simulink model "stabilization_model"  (R2024b)
settings: Solver=ode4  StartTime=0.0  StopTime=30  FixedStep=0.0001  MaxStep=0.0005  RelTol=1e-5
values from neighbouring files (symbols this model uses):
  B_m = 0.0015    [model_consts.m]
  Bmh = 0.0015    [model_consts.m]
  C1 = 10e4    (= 100000)    [model_consts.m]
  C2 = 3    [model_consts.m]
  f_const = (4*pi^2*ni*N^2*l_1*l_2)/(p_h^2)    (= 461404.005751)    [model_consts.m]
  g1_const = (2*k_t*pi*ni*N)/(p_h*R)    (= 6268.81826761)    [model_consts.m]
  g3_const = f_const*(k_t*k_e)/(R+B_m)    (= 1536817.32754)    [model_consts.m]
  g4_const = f_const*J_m    (= 922.808011502)    [model_consts.m]
  J = 3400    [model_consts.m]
  J_m = 0.002    [model_consts.m]
  Jh = J_w + J_a + J_mw*nih*R_z*(1/R_w)    (= 26100.0000385)    [model_consts.m]
  kh_e = 0.401    [model_consts.m]
  kh_t = 0.54    [model_consts.m]
  l_1 = 0.32    [model_consts.m]
  l_2 = 0.44    [model_consts.m]
  mg = m*g    (= 19620)    [model_consts.m]
  mgl = m*g*l    (= 2354.4)    [model_consts.m]
  mwag = g*(mw+ma)    (= 186390)    [model_consts.m]
  nih = 0.97    [model_consts.m]
  q_0 = acos((l_1^2+l_2^2-l_0^2)/(2*l_1*l_2))    [model_consts.m]
  R_h = 0.01437    [model_consts.m]
  r_t = 0.05    [model_consts.m]
  R_w = 1.2    [model_consts.m]
  R_z = 0.08    [model_consts.m]
  u_k = 0.04    [model_consts.m]
  u_s = 0.12    [model_consts.m]
  uw_k = 0.0015    [model_consts.m]
  uw_s = 0.0025    [model_consts.m]
libraries: slpidlib x6, SignalEditorBlockLib x1
settings Model: Creator=ksapi  LastModifiedBy=ksapi

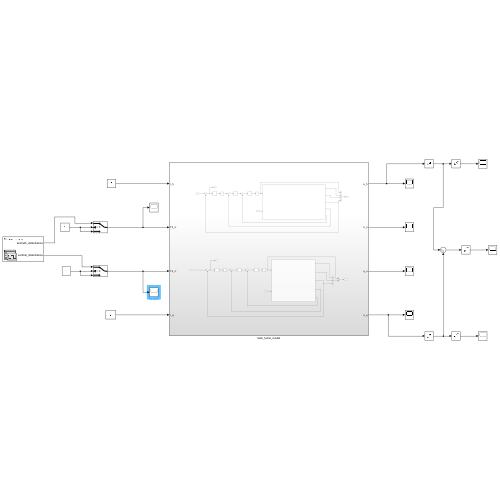
[thumbnail: Simulink's stored preview of the top-level diagram]
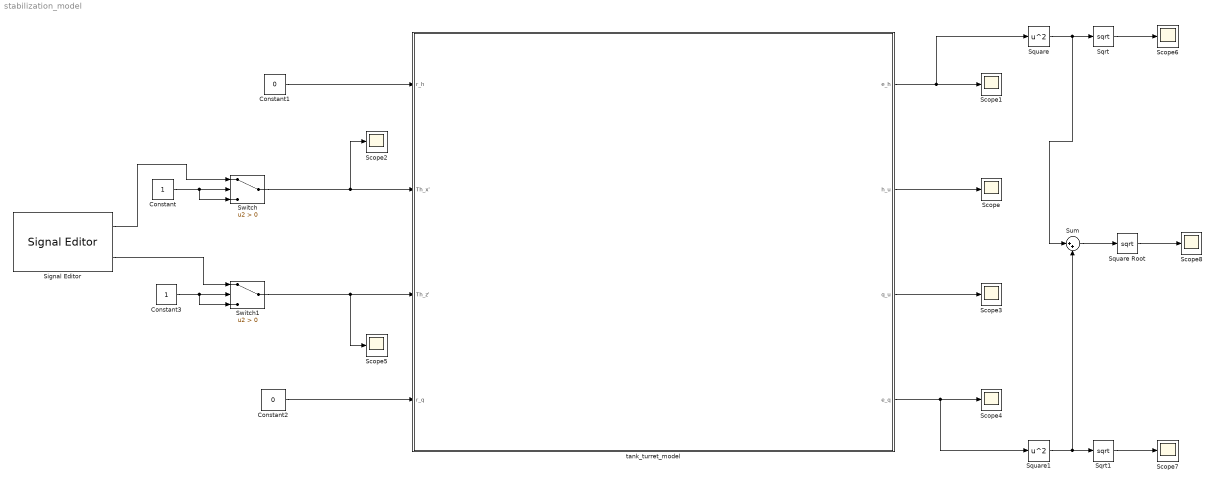
== system stabilization_model ==
  Constant : Constant
  Constant1 : Constant  Value=0
  Constant2 : Constant  Value=0
  Constant3 : Constant
  Scope{,1..8} (9 alike) : Scope
  Signal Editor : SignalEditorBlockLib/Signal Editor  FileName=disturbance_scenarios.mat  ActiveScenario=Sinous_course  ActiveSignal=azimuth_disturbance  IsBus=off  OutputBusObjectStr=Bus: BusObject  SampleTime=0  Interpolate=off  ZeroCross=off  OutputAfterFinalValue=Setting to zero  Unit=inherit  PreserveSignalName=on  ApplySigPropsToAllScenarios=on  ApplySigPropsToAllSignals=off
  Sqrt : Sqrt
  Sqrt1 : Sqrt
  Square : Math  Operator=square
  Square Root : Sqrt
  Square1 : Math  Operator=square
  Sum : Sum  Inputs=|++
  Switch : Switch  Criteria=u2 > Threshold  SaturateOnIntegerOverflow=off  InputSameDT=off
  Switch1 : Switch  Criteria=u2 > Threshold  SaturateOnIntegerOverflow=off  InputSameDT=off
  tank_turret_model : Subsystem
  wires:
  Constant1/1 -> tank_turret_model/1(r_h)
  Signal Editor/2 -> Switch1/1
  Constant2/1 -> tank_turret_model/4(r_q)
  tank_turret_model/1(e_h) -> Square/1, Scope1/1
  tank_turret_model/2(h_u) -> Scope/1
  tank_turret_model/3(q_u) -> Scope3/1
  Square/1 -> Sum/1, Sqrt/1
  Sqrt/1 -> Scope6/1
  Constant/1 -> Switch/3, Switch/2
  Constant3/1 -> Switch1/3, Switch1/2
  Signal Editor/1 -> Switch/1
  Square1/1 -> Sqrt1/1, Sum/2
  Sqrt1/1 -> Scope7/1
  tank_turret_model/4(e_q) -> Square1/1, Scope4/1
  Sum/1 -> Square Root/1
  Square Root/1 -> Scope8/1
  Switch/1 -> tank_turret_model/2(Th_x'), Scope2/1
  Switch1/1 -> tank_turret_model/3(Th_z'), Scope5/1

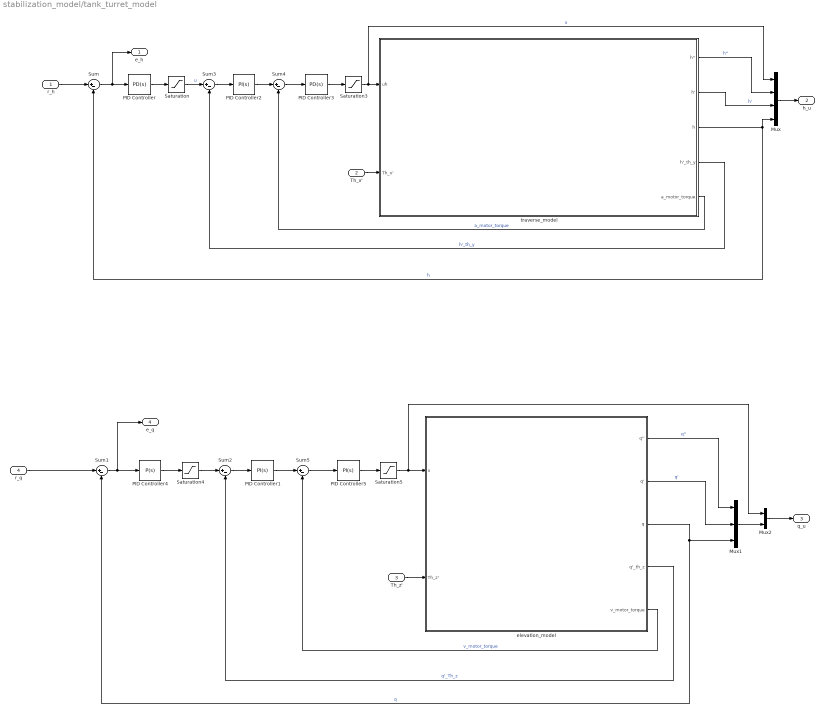
== system stabilization_model/tank_turret_model ==
  r_h : Inport
  Th_x' : Inport  Port=2
  Th_z' : Inport  Port=3
  r_q : Inport  Port=4
  Mux : Mux
  Mux1 : Mux  Inputs=3
  Mux2 : Mux  Inputs=2
  PID Controller : slpidlib/PID Controller  Controller=PD  Form=Parallel  TimeDomain=Continuous-time  UseExternalTs=off  SampleTime=-1  IntegratorMethod=Forward Euler  FilterMethod=Forward Euler  ControllerParametersSource=internal  P=140  I=0  UseKiTs=off  D=90  UseExternalDerivativeSource=off  N=100  UseFilter=on  TunerSelectOption=Transfer Function Based (PID Tuner App)  InitialConditionSource=internal  InitialConditionForIntegrator=0  InitialConditionForFilter=0  DifferentiatorICPrevScaledInput=0  ExternalReset=none  TrackingMode=off  Kt=1  LimitOutput=off  SatLimitsSource=internal  UpperSaturationLimit=inf  LowerSaturationLimit=-inf  LinearizeAsGain=on  AntiWindupMode=none  Kb=1  LimitIntegrator=off  UpperIntegratorSaturationLimit=inf  LowerIntegratorSaturationLimit=-inf  POutMin=[]  POutMax=[]  IOutMin=[]  IOutMax=[]  DOutMin=[]  DOutMax=[]  NOutMin=[]  NOutMax=[]  SumOutMin=[]  SumOutMax=[]  SaturationOutMin=[]  SaturationOutMax=[]  PParamMin=[]  PParamMax=[]  IParamMin=[]  IParamMax=[]  DParamMin=[]  DParamMax=[]  NParamMin=[]  NParamMax=[]  KbParamMin=[]  KbParamMax=[]  KtParamMin=[]  KtParamMax=[]  KbOutMin=[]  KbOutMax=[]  KtOutMin=[]  KtOutMax=[]  IntegratorOutMin=[]  IntegratorOutMax=[]  FilterOutMin=[]  FilterOutMax=[]  SumI1OutMin=[]  SumI1OutMax=[]  SumI2OutMin=[]  SumI2OutMax=[]  SumI3OutMin=[]  SumI3OutMax=[]  SumI4OutMin=[]  SumI4OutMax=[]  SumDOutMin=[]  SumDOutMax=[]  DifferentiatorOutMin=[]  DifferentiatorOutMax=[]  FilterDiffOutCoefMin=[]  FilterDiffOutCoefMax=[]  ReciprocalOutMin=[]  ReciprocalOutMax=[]  SumDenOutMin=[]  SumDenOutMax=[]  SumNumOutMin=[]  SumNumOutMax=[]  DivideOutMin=[]  DivideOutMax=[]  UdiffTsProdOutMin=[]  UdiffTsProdOutMax=[]  NTsProdOutMin=[]  NTsProdOutMax=[]  UintegralTsProdOutMin=[]  UintegralTsProdOutMax=[]  UngainTsProdOutMin=[]  UngainTsProdOutMax=[]  ClampingZeroOutDataTypeStr=Inherit: Inherit via back propagation  ClampingZeroOutMin=[]  ClampingZeroOutMax=[]  FilterDenConstantOutDataTypeStr=Inherit: Inherit via back propagation  FilterDenConstantOutMin=[]  FilterDenConstantOutMax=[]  PCopyOutDataTypeStr=Inherit: Inherit via back propagation  PCopyOutMin=[]  PCopyOutMax=[]  NCopyOutDataTypeStr=Inherit: Inherit via back propagation  NCopyOutMin=[]  NCopyOutMax=[]  IntegratorContinuousStateAttributes=''  IntegratorStateMustResolveToSignalObject=off  IntegratorRTWStateStorageClass=Auto  FilterContinuousStateAttributes=''  FilterStateMustResolveToSignalObject=off  FilterRTWStateStorageClass=Auto  ParallelPVariant=InternalParameters  IdealPVariant=Disabled  IVariant=Disabled  DVariant=InternalParameters  IntegratorVariant=Disabled  SatVariant=Disabled  AWVariant=Disabled  PCopyVariant=Disabled  TRVariant=Disabled  FdbkBlocksVariant=Forward  IdealPFdbkVariant=Disabled  SatFdbkVariant=Disabled  DerivativeFilterVariant=ContFilter  NVariant=InternalParameters  NCopyVariant=Disabled  FilterICVariant=InternalICsFilter  IntegratorICVariant=Disabled  ExternalResetVariant=Disabled  TRSumVariant=Passthrough  SumFdbkVariant=Disabled  SumVariant=Sum_PD  TsampFilterVariant=InternalTs  TsampNgainVariant=Passthrough  TsampIntegralVariant=Disabled_SignalSpec  ExternalSaturationOutDataTypeStr=Inherit: Same as second input  DerivativeSourceVariant=ErrorSignal  PreIntVariant=InternalPreInt
  PID Controller1 : slpidlib/PID Controller  Controller=PI  Form=Parallel  TimeDomain=Continuous-time  UseExternalTs=off  SampleTime=-1  IntegratorMethod=Forward Euler  FilterMethod=Forward Euler  ControllerParametersSource=internal  P=1250  I=1000  UseKiTs=off  D=5  UseExternalDerivativeSource=off  N=100  UseFilter=on  TunerSelectOption=Transfer Function Based (PID Tuner App)  InitialConditionSource=internal  InitialConditionForIntegrator=0  InitialConditionForFilter=0  DifferentiatorICPrevScaledInput=0  ExternalReset=none  TrackingMode=off  Kt=1  LimitOutput=off  SatLimitsSource=internal  UpperSaturationLimit=inf  LowerSaturationLimit=-inf  LinearizeAsGain=on  AntiWindupMode=none  Kb=1  LimitIntegrator=off  UpperIntegratorSaturationLimit=inf  LowerIntegratorSaturationLimit=-inf  POutMin=[]  POutMax=[]  IOutMin=[]  IOutMax=[]  DOutMin=[]  DOutMax=[]  NOutMin=[]  NOutMax=[]  SumOutMin=[]  SumOutMax=[]  SaturationOutMin=[]  SaturationOutMax=[]  PParamMin=[]  PParamMax=[]  IParamMin=[]  IParamMax=[]  DParamMin=[]  DParamMax=[]  NParamMin=[]  NParamMax=[]  KbParamMin=[]  KbParamMax=[]  KtParamMin=[]  KtParamMax=[]  KbOutMin=[]  KbOutMax=[]  KtOutMin=[]  KtOutMax=[]  IntegratorOutMin=[]  IntegratorOutMax=[]  FilterOutMin=[]  FilterOutMax=[]  SumI1OutMin=[]  SumI1OutMax=[]  SumI2OutMin=[]  SumI2OutMax=[]  SumI3OutMin=[]  SumI3OutMax=[]  SumI4OutMin=[]  SumI4OutMax=[]  SumDOutMin=[]  SumDOutMax=[]  DifferentiatorOutMin=[]  DifferentiatorOutMax=[]  FilterDiffOutCoefMin=[]  FilterDiffOutCoefMax=[]  ReciprocalOutMin=[]  ReciprocalOutMax=[]  SumDenOutMin=[]  SumDenOutMax=[]  SumNumOutMin=[]  SumNumOutMax=[]  DivideOutMin=[]  DivideOutMax=[]  UdiffTsProdOutMin=[]  UdiffTsProdOutMax=[]  NTsProdOutMin=[]  NTsProdOutMax=[]  UintegralTsProdOutMin=[]  UintegralTsProdOutMax=[]  UngainTsProdOutMin=[]  UngainTsProdOutMax=[]  ClampingZeroOutDataTypeStr=Inherit: Inherit via back propagation  ClampingZeroOutMin=[]  ClampingZeroOutMax=[]  FilterDenConstantOutDataTypeStr=Inherit: Inherit via back propagation  FilterDenConstantOutMin=[]  FilterDenConstantOutMax=[]  PCopyOutDataTypeStr=Inherit: Inherit via back propagation  PCopyOutMin=[]  PCopyOutMax=[]  NCopyOutDataTypeStr=Inherit: Inherit via back propagation  NCopyOutMin=[]  NCopyOutMax=[]  IntegratorContinuousStateAttributes=''  IntegratorStateMustResolveToSignalObject=off  IntegratorRTWStateStorageClass=Auto  FilterContinuousStateAttributes=''  FilterStateMustResolveToSignalObject=off  FilterRTWStateStorageClass=Auto  ParallelPVariant=InternalParameters  IdealPVariant=Disabled  IVariant=InternalParameters  DVariant=Disabled  IntegratorVariant=Continuous  SatVariant=Disabled  AWVariant=Passthrough  PCopyVariant=Disabled  TRVariant=Disabled  FdbkBlocksVariant=Forward  IdealPFdbkVariant=Disabled  SatFdbkVariant=Disabled  DerivativeFilterVariant=Disabled  NVariant=Disabled  NCopyVariant=Disabled_SignalSpec  FilterICVariant=Disabled  IntegratorICVariant=InternalICs  ExternalResetVariant=Disabled  TRSumVariant=Passthrough  SumFdbkVariant=Disabled  SumVariant=Sum_PI  TsampFilterVariant=InternalTs  TsampNgainVariant=Passthrough  TsampIntegralVariant=Disabled_SignalSpec  ExternalSaturationOutDataTypeStr=Inherit: Same as second input  DerivativeSourceVariant=Disabled  PreIntVariant=InternalPreInt
  PID Controller2 : slpidlib/PID Controller  Controller=PI  Form=Parallel  TimeDomain=Continuous-time  UseExternalTs=off  SampleTime=-1  IntegratorMethod=Forward Euler  FilterMethod=Forward Euler  ControllerParametersSource=internal  P=100000  I=125000  UseKiTs=off  D=0  UseExternalDerivativeSource=off  N=100  UseFilter=on  TunerSelectOption=Transfer Function Based (PID Tuner App)  InitialConditionSource=internal  InitialConditionForIntegrator=0  InitialConditionForFilter=0  DifferentiatorICPrevScaledInput=0  ExternalReset=none  TrackingMode=off  Kt=1  LimitOutput=off  SatLimitsSource=internal  UpperSaturationLimit=inf  LowerSaturationLimit=-inf  LinearizeAsGain=on  AntiWindupMode=none  Kb=1  LimitIntegrator=off  UpperIntegratorSaturationLimit=inf  LowerIntegratorSaturationLimit=-inf  POutMin=[]  POutMax=[]  IOutMin=[]  IOutMax=[]  DOutMin=[]  DOutMax=[]  NOutMin=[]  NOutMax=[]  SumOutMin=[]  SumOutMax=[]  SaturationOutMin=[]  SaturationOutMax=[]  PParamMin=[]  PParamMax=[]  IParamMin=[]  IParamMax=[]  DParamMin=[]  DParamMax=[]  NParamMin=[]  NParamMax=[]  KbParamMin=[]  KbParamMax=[]  KtParamMin=[]  KtParamMax=[]  KbOutMin=[]  KbOutMax=[]  KtOutMin=[]  KtOutMax=[]  IntegratorOutMin=[]  IntegratorOutMax=[]  FilterOutMin=[]  FilterOutMax=[]  SumI1OutMin=[]  SumI1OutMax=[]  SumI2OutMin=[]  SumI2OutMax=[]  SumI3OutMin=[]  SumI3OutMax=[]  SumI4OutMin=[]  SumI4OutMax=[]  SumDOutMin=[]  SumDOutMax=[]  DifferentiatorOutMin=[]  DifferentiatorOutMax=[]  FilterDiffOutCoefMin=[]  FilterDiffOutCoefMax=[]  ReciprocalOutMin=[]  ReciprocalOutMax=[]  SumDenOutMin=[]  SumDenOutMax=[]  SumNumOutMin=[]  SumNumOutMax=[]  DivideOutMin=[]  DivideOutMax=[]  UdiffTsProdOutMin=[]  UdiffTsProdOutMax=[]  NTsProdOutMin=[]  NTsProdOutMax=[]  UintegralTsProdOutMin=[]  UintegralTsProdOutMax=[]  UngainTsProdOutMin=[]  UngainTsProdOutMax=[]  ClampingZeroOutDataTypeStr=Inherit: Inherit via back propagation  ClampingZeroOutMin=[]  ClampingZeroOutMax=[]  FilterDenConstantOutDataTypeStr=Inherit: Inherit via back propagation  FilterDenConstantOutMin=[]  FilterDenConstantOutMax=[]  PCopyOutDataTypeStr=Inherit: Inherit via back propagation  PCopyOutMin=[]  PCopyOutMax=[]  NCopyOutDataTypeStr=Inherit: Inherit via back propagation  NCopyOutMin=[]  NCopyOutMax=[]  IntegratorContinuousStateAttributes=''  IntegratorStateMustResolveToSignalObject=off  IntegratorRTWStateStorageClass=Auto  FilterContinuousStateAttributes=''  FilterStateMustResolveToSignalObject=off  FilterRTWStateStorageClass=Auto  ParallelPVariant=InternalParameters  IdealPVariant=Disabled  IVariant=InternalParameters  DVariant=Disabled  IntegratorVariant=Continuous  SatVariant=Disabled  AWVariant=Passthrough  PCopyVariant=Disabled  TRVariant=Disabled  FdbkBlocksVariant=Forward  IdealPFdbkVariant=Disabled  SatFdbkVariant=Disabled  DerivativeFilterVariant=Disabled  NVariant=Disabled  NCopyVariant=Disabled_SignalSpec  FilterICVariant=Disabled  IntegratorICVariant=InternalICs  ExternalResetVariant=Disabled  TRSumVariant=Passthrough  SumFdbkVariant=Disabled  SumVariant=Sum_PI  TsampFilterVariant=InternalTs  TsampNgainVariant=Passthrough  TsampIntegralVariant=Disabled_SignalSpec  ExternalSaturationOutDataTypeStr=Inherit: Same as second input  DerivativeSourceVariant=Disabled  PreIntVariant=InternalPreInt
  PID Controller3 : slpidlib/PID Controller  Controller=PD  Form=Parallel  TimeDomain=Continuous-time  UseExternalTs=off  SampleTime=-1  IntegratorMethod=Forward Euler  FilterMethod=Forward Euler  ControllerParametersSource=internal  P=0.5  I=10  UseKiTs=off  D=0.1  UseExternalDerivativeSource=off  N=100  UseFilter=on  TunerSelectOption=Transfer Function Based (PID Tuner App)  InitialConditionSource=internal  InitialConditionForIntegrator=0  InitialConditionForFilter=0  DifferentiatorICPrevScaledInput=0  ExternalReset=none  TrackingMode=off  Kt=1  LimitOutput=off  SatLimitsSource=internal  UpperSaturationLimit=inf  LowerSaturationLimit=-inf  LinearizeAsGain=on  AntiWindupMode=none  Kb=1  LimitIntegrator=off  UpperIntegratorSaturationLimit=inf  LowerIntegratorSaturationLimit=-inf  POutMin=[]  POutMax=[]  IOutMin=[]  IOutMax=[]  DOutMin=[]  DOutMax=[]  NOutMin=[]  NOutMax=[]  SumOutMin=[]  SumOutMax=[]  SaturationOutMin=[]  SaturationOutMax=[]  PParamMin=[]  PParamMax=[]  IParamMin=[]  IParamMax=[]  DParamMin=[]  DParamMax=[]  NParamMin=[]  NParamMax=[]  KbParamMin=[]  KbParamMax=[]  KtParamMin=[]  KtParamMax=[]  KbOutMin=[]  KbOutMax=[]  KtOutMin=[]  KtOutMax=[]  IntegratorOutMin=[]  IntegratorOutMax=[]  FilterOutMin=[]  FilterOutMax=[]  SumI1OutMin=[]  SumI1OutMax=[]  SumI2OutMin=[]  SumI2OutMax=[]  SumI3OutMin=[]  SumI3OutMax=[]  SumI4OutMin=[]  SumI4OutMax=[]  SumDOutMin=[]  SumDOutMax=[]  DifferentiatorOutMin=[]  DifferentiatorOutMax=[]  FilterDiffOutCoefMin=[]  FilterDiffOutCoefMax=[]  ReciprocalOutMin=[]  ReciprocalOutMax=[]  SumDenOutMin=[]  SumDenOutMax=[]  SumNumOutMin=[]  SumNumOutMax=[]  DivideOutMin=[]  DivideOutMax=[]  UdiffTsProdOutMin=[]  UdiffTsProdOutMax=[]  NTsProdOutMin=[]  NTsProdOutMax=[]  UintegralTsProdOutMin=[]  UintegralTsProdOutMax=[]  UngainTsProdOutMin=[]  UngainTsProdOutMax=[]  ClampingZeroOutDataTypeStr=Inherit: Inherit via back propagation  ClampingZeroOutMin=[]  ClampingZeroOutMax=[]  FilterDenConstantOutDataTypeStr=Inherit: Inherit via back propagation  FilterDenConstantOutMin=[]  FilterDenConstantOutMax=[]  PCopyOutDataTypeStr=Inherit: Inherit via back propagation  PCopyOutMin=[]  PCopyOutMax=[]  NCopyOutDataTypeStr=Inherit: Inherit via back propagation  NCopyOutMin=[]  NCopyOutMax=[]  IntegratorContinuousStateAttributes=''  IntegratorStateMustResolveToSignalObject=off  IntegratorRTWStateStorageClass=Auto  FilterContinuousStateAttributes=''  FilterStateMustResolveToSignalObject=off  FilterRTWStateStorageClass=Auto  ParallelPVariant=InternalParameters  IdealPVariant=Disabled  IVariant=Disabled  DVariant=InternalParameters  IntegratorVariant=Disabled  SatVariant=Disabled  AWVariant=Disabled  PCopyVariant=Disabled  TRVariant=Disabled  FdbkBlocksVariant=Forward  IdealPFdbkVariant=Disabled  SatFdbkVariant=Disabled  DerivativeFilterVariant=ContFilter  NVariant=InternalParameters  NCopyVariant=Disabled  FilterICVariant=InternalICsFilter  IntegratorICVariant=Disabled  ExternalResetVariant=Disabled  TRSumVariant=Passthrough  SumFdbkVariant=Disabled  SumVariant=Sum_PD  TsampFilterVariant=InternalTs  TsampNgainVariant=Passthrough  TsampIntegralVariant=Disabled_SignalSpec  ExternalSaturationOutDataTypeStr=Inherit: Same as second input  DerivativeSourceVariant=ErrorSignal  PreIntVariant=InternalPreInt
  PID Controller4 : slpidlib/PID Controller  Controller=P  Form=Parallel  TimeDomain=Continuous-time  UseExternalTs=off  SampleTime=-1  IntegratorMethod=Forward Euler  FilterMethod=Forward Euler  ControllerParametersSource=internal  P=500  I=0  UseKiTs=off  D=0  UseExternalDerivativeSource=off  N=100  UseFilter=on  TunerSelectOption=Transfer Function Based (PID Tuner App)  InitialConditionSource=internal  InitialConditionForIntegrator=0  InitialConditionForFilter=0  DifferentiatorICPrevScaledInput=0  ExternalReset=none  TrackingMode=off  Kt=1  LimitOutput=off  SatLimitsSource=internal  UpperSaturationLimit=inf  LowerSaturationLimit=-inf  LinearizeAsGain=on  AntiWindupMode=none  Kb=1  LimitIntegrator=off  UpperIntegratorSaturationLimit=inf  LowerIntegratorSaturationLimit=-inf  POutMin=[]  POutMax=[]  IOutMin=[]  IOutMax=[]  DOutMin=[]  DOutMax=[]  NOutMin=[]  NOutMax=[]  SumOutMin=[]  SumOutMax=[]  SaturationOutMin=[]  SaturationOutMax=[]  PParamMin=[]  PParamMax=[]  IParamMin=[]  IParamMax=[]  DParamMin=[]  DParamMax=[]  NParamMin=[]  NParamMax=[]  KbParamMin=[]  KbParamMax=[]  KtParamMin=[]  KtParamMax=[]  KbOutMin=[]  KbOutMax=[]  KtOutMin=[]  KtOutMax=[]  IntegratorOutMin=[]  IntegratorOutMax=[]  FilterOutMin=[]  FilterOutMax=[]  SumI1OutMin=[]  SumI1OutMax=[]  SumI2OutMin=[]  SumI2OutMax=[]  SumI3OutMin=[]  SumI3OutMax=[]  SumI4OutMin=[]  SumI4OutMax=[]  SumDOutMin=[]  SumDOutMax=[]  DifferentiatorOutMin=[]  DifferentiatorOutMax=[]  FilterDiffOutCoefMin=[]  FilterDiffOutCoefMax=[]  ReciprocalOutMin=[]  ReciprocalOutMax=[]  SumDenOutMin=[]  SumDenOutMax=[]  SumNumOutMin=[]  SumNumOutMax=[]  DivideOutMin=[]  DivideOutMax=[]  UdiffTsProdOutMin=[]  UdiffTsProdOutMax=[]  NTsProdOutMin=[]  NTsProdOutMax=[]  UintegralTsProdOutMin=[]  UintegralTsProdOutMax=[]  UngainTsProdOutMin=[]  UngainTsProdOutMax=[]  ClampingZeroOutDataTypeStr=Inherit: Inherit via back propagation  ClampingZeroOutMin=[]  ClampingZeroOutMax=[]  FilterDenConstantOutDataTypeStr=Inherit: Inherit via back propagation  FilterDenConstantOutMin=[]  FilterDenConstantOutMax=[]  PCopyOutDataTypeStr=Inherit: Inherit via back propagation  PCopyOutMin=[]  PCopyOutMax=[]  NCopyOutDataTypeStr=Inherit: Inherit via back propagation  NCopyOutMin=[]  NCopyOutMax=[]  IntegratorContinuousStateAttributes=''  IntegratorStateMustResolveToSignalObject=off  IntegratorRTWStateStorageClass=Auto  FilterContinuousStateAttributes=''  FilterStateMustResolveToSignalObject=off  FilterRTWStateStorageClass=Auto  ParallelPVariant=InternalParameters  IdealPVariant=Disabled  IVariant=Disabled  DVariant=Disabled  IntegratorVariant=Disabled  SatVariant=Disabled  AWVariant=Disabled  PCopyVariant=Disabled  TRVariant=Disabled  FdbkBlocksVariant=Forward  IdealPFdbkVariant=Disabled  SatFdbkVariant=Disabled  DerivativeFilterVariant=Disabled  NVariant=Disabled  NCopyVariant=Disabled_SignalSpec  FilterICVariant=Disabled  IntegratorICVariant=Disabled  ExternalResetVariant=Disabled  TRSumVariant=Passthrough  SumFdbkVariant=Disabled  SumVariant=Passthrough_P  TsampFilterVariant=InternalTs  TsampNgainVariant=Passthrough  TsampIntegralVariant=Disabled_SignalSpec  ExternalSaturationOutDataTypeStr=Inherit: Same as second input  DerivativeSourceVariant=Disabled  PreIntVariant=InternalPreInt
  PID Controller5 : slpidlib/PID Controller  Controller=PI  Form=Parallel  TimeDomain=Continuous-time  UseExternalTs=off  SampleTime=-1  IntegratorMethod=Forward Euler  FilterMethod=Forward Euler  ControllerParametersSource=internal  P=5  I=3  UseKiTs=off  D=0  UseExternalDerivativeSource=off  N=100  UseFilter=on  TunerSelectOption=Transfer Function Based (PID Tuner App)  InitialConditionSource=internal  InitialConditionForIntegrator=0  InitialConditionForFilter=0  DifferentiatorICPrevScaledInput=0  ExternalReset=none  TrackingMode=off  Kt=1  LimitOutput=off  SatLimitsSource=internal  UpperSaturationLimit=inf  LowerSaturationLimit=-inf  LinearizeAsGain=on  AntiWindupMode=none  Kb=1  LimitIntegrator=off  UpperIntegratorSaturationLimit=inf  LowerIntegratorSaturationLimit=-inf  POutMin=[]  POutMax=[]  IOutMin=[]  IOutMax=[]  DOutMin=[]  DOutMax=[]  NOutMin=[]  NOutMax=[]  SumOutMin=[]  SumOutMax=[]  SaturationOutMin=[]  SaturationOutMax=[]  PParamMin=[]  PParamMax=[]  IParamMin=[]  IParamMax=[]  DParamMin=[]  DParamMax=[]  NParamMin=[]  NParamMax=[]  KbParamMin=[]  KbParamMax=[]  KtParamMin=[]  KtParamMax=[]  KbOutMin=[]  KbOutMax=[]  KtOutMin=[]  KtOutMax=[]  IntegratorOutMin=[]  IntegratorOutMax=[]  FilterOutMin=[]  FilterOutMax=[]  SumI1OutMin=[]  SumI1OutMax=[]  SumI2OutMin=[]  SumI2OutMax=[]  SumI3OutMin=[]  SumI3OutMax=[]  SumI4OutMin=[]  SumI4OutMax=[]  SumDOutMin=[]  SumDOutMax=[]  DifferentiatorOutMin=[]  DifferentiatorOutMax=[]  FilterDiffOutCoefMin=[]  FilterDiffOutCoefMax=[]  ReciprocalOutMin=[]  ReciprocalOutMax=[]  SumDenOutMin=[]  SumDenOutMax=[]  SumNumOutMin=[]  SumNumOutMax=[]  DivideOutMin=[]  DivideOutMax=[]  UdiffTsProdOutMin=[]  UdiffTsProdOutMax=[]  NTsProdOutMin=[]  NTsProdOutMax=[]  UintegralTsProdOutMin=[]  UintegralTsProdOutMax=[]  UngainTsProdOutMin=[]  UngainTsProdOutMax=[]  ClampingZeroOutDataTypeStr=Inherit: Inherit via back propagation  ClampingZeroOutMin=[]  ClampingZeroOutMax=[]  FilterDenConstantOutDataTypeStr=Inherit: Inherit via back propagation  FilterDenConstantOutMin=[]  FilterDenConstantOutMax=[]  PCopyOutDataTypeStr=Inherit: Inherit via back propagation  PCopyOutMin=[]  PCopyOutMax=[]  NCopyOutDataTypeStr=Inherit: Inherit via back propagation  NCopyOutMin=[]  NCopyOutMax=[]  IntegratorContinuousStateAttributes=''  IntegratorStateMustResolveToSignalObject=off  IntegratorRTWStateStorageClass=Auto  FilterContinuousStateAttributes=''  FilterStateMustResolveToSignalObject=off  FilterRTWStateStorageClass=Auto  ParallelPVariant=InternalParameters  IdealPVariant=Disabled  IVariant=InternalParameters  DVariant=Disabled  IntegratorVariant=Continuous  SatVariant=Disabled  AWVariant=Passthrough  PCopyVariant=Disabled  TRVariant=Disabled  FdbkBlocksVariant=Forward  IdealPFdbkVariant=Disabled  SatFdbkVariant=Disabled  DerivativeFilterVariant=Disabled  NVariant=Disabled  NCopyVariant=Disabled_SignalSpec  FilterICVariant=Disabled  IntegratorICVariant=InternalICs  ExternalResetVariant=Disabled  TRSumVariant=Passthrough  SumFdbkVariant=Disabled  SumVariant=Sum_PI  TsampFilterVariant=InternalTs  TsampNgainVariant=Passthrough  TsampIntegralVariant=Disabled_SignalSpec  ExternalSaturationOutDataTypeStr=Inherit: Same as second input  DerivativeSourceVariant=Disabled  PreIntVariant=InternalPreInt
  Saturation : Saturate  UpperLimit=0.75  LowerLimit=-0.75
  Saturation3 : Saturate  UpperLimit=270  LowerLimit=-270
  Saturation4 : Saturate  UpperLimit=0.15  LowerLimit=-0.15
  Saturation5 : Saturate  UpperLimit=270  LowerLimit=-270
  Sum{,1..5} (6 alike) : Sum  Inputs=|+-
  elevation_model : Subsystem
  traverse_model : Subsystem
  e_h : Outport
  h_u : Outport  Port=2
  q_u : Outport  Port=3
  e_q : Outport  Port=4
  wires:
  Mux/1 -> h_u/1
  elevation_model/3(q) -> Sum1/2, Mux1/3  "q"
  traverse_model/1(h'') -> Mux/2  "h''"
  elevation_model/2(q') -> Mux1/2  "q'"
  traverse_model/2(h') -> Mux/3  "h'"
  PID Controller/1 -> Saturation/1
  Mux1/1 -> Mux2/2
  traverse_model/3(h) -> Sum/2, Mux/4  "h"
  Sum/1 -> PID Controller/1, e_h/1
  elevation_model/1(q'') -> Mux1/1  "q''"
  r_h/1 -> Sum/1
  Sum1/1 -> e_q/1, PID Controller4/1
  Mux2/1 -> q_u/1
  Th_z'/1 -> elevation_model/2(Th_z')
  elevation_model/4(q'_th_z) -> Sum2/2  "q'_Th_z"
  Th_x'/1 -> traverse_model/2(Th_x')
  PID Controller1/1 -> Sum5/1
  Saturation/1 -> Sum3/1  "u"
  Sum2/1 -> PID Controller1/1
  Sum3/1 -> PID Controller2/1
  traverse_model/4(h'_th_y) -> Sum3/2  "h'_th_y"
  PID Controller2/1 -> Sum4/1
  PID Controller3/1 -> Saturation3/1
  Sum4/1 -> PID Controller3/1
  traverse_model/5(a_motor_torque) -> Sum4/2  "a_motor_torque"
  Saturation3/1 -> traverse_model/1(uh), Mux/1  "u"
  PID Controller4/1 -> Saturation4/1
  Saturation4/1 -> Sum2/1
  PID Controller5/1 -> Saturation5/1
  Sum5/1 -> PID Controller5/1
  Saturation5/1 -> Mux2/1, elevation_model/1(u)
  elevation_model/5(v_motor_torque) -> Sum5/2  "v_motor_torque"
  r_q/1 -> Sum1/1

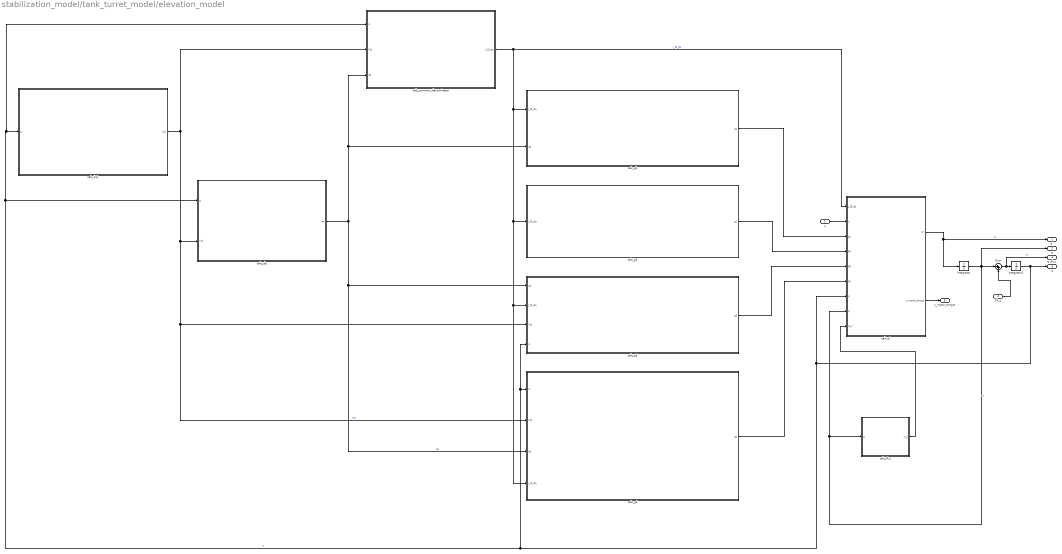
== system stabilization_model/tank_turret_model/elevation_model ==
  u : Inport
  Th_z' : Inport  Port=2
  Integrator : Integrator
  Integrator1 : Integrator
  Sum : Sum  Inputs=|++
  calc_M_t : Subsystem
  calc_common_denominator : Subsystem
  calc_dq : Subsystem
  calc_g1 : Subsystem
  calc_g2 : Subsystem
  calc_g3 : Subsystem
  calc_g4 : Subsystem
  calc_l(q) : Subsystem
  calc_q'' : Subsystem
  q'' : Outport
  q' : Outport  Port=2
  q : Outport  Port=3
  q'_th_z : Outport  Port=4
  v_motor_torque : Outport  Port=5
  wires:
  calc_q''/1(q'') -> Integrator/1, q''/1  "q''"
  calc_g4/1(g4) -> calc_q''/6(g4)
  calc_dq/1(dq) -> calc_common_denominator/3(dq), calc_g1/2(dq), calc_g4/3(dq), calc_g3/1(dq)  "dq"
  u/1 -> calc_q''/2(u)
  calc_l(q)/1(l(q)) -> calc_g4/2(l(q)), calc_g3/3(l(q)), calc_dq/2(l(q)), calc_common_denominator/2(l(q))  "l(q)"
  calc_g3/1(g3) -> calc_q''/5(g3)
  calc_common_denominator/1(J_f3_dq) -> calc_q''/1(J_f3_dq), calc_g4/4(J_f3_dq), calc_g3/2(J_f3_dq), calc_g2/1(J_f3_dq), calc_g1/1(J_f3_dq)  "J_f3_dq"
  calc_g1/1(g1) -> calc_q''/3(g1)
  calc_g2/1(g2) -> calc_q''/4(g2)
  Integrator/1 -> q'/1, Sum/1, calc_q''/8(q'), calc_M_t/1(q')  "q'"
  Integrator1/1 -> calc_dq/1(q), calc_l(q)/1(q), calc_common_denominator/1(q), calc_g3/4(q), calc_g4/1(q), calc_q''/7(q), q/1  "q"
  calc_M_t/1(M_t) -> calc_q''/9(M_t)
  Th_z'/1 -> Sum/2
  Sum/1 -> q'_th_z/1, Integrator1/1  "q'"
  calc_q''/2(v_motor_torque) -> v_motor_torque/1

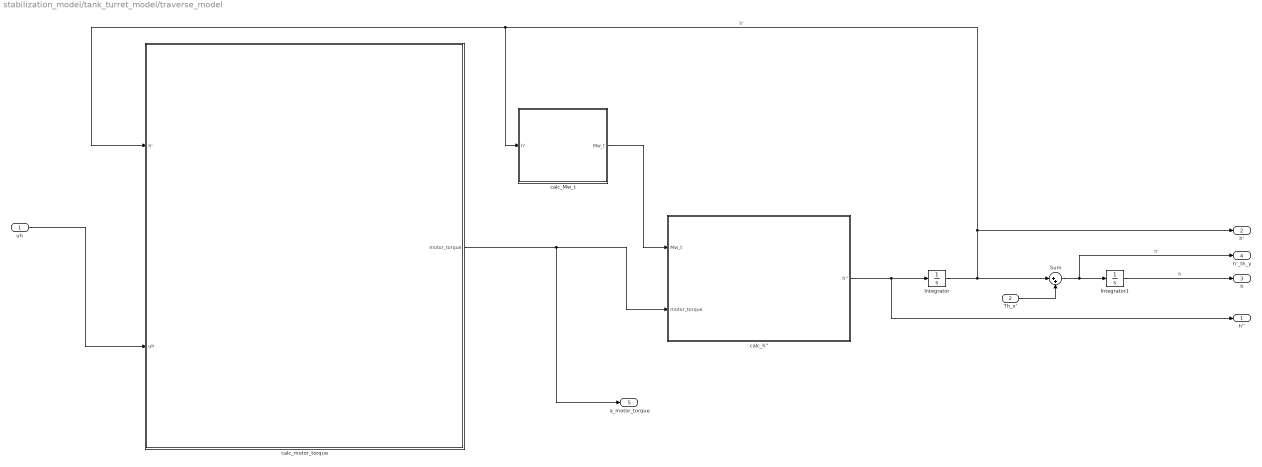
== system stabilization_model/tank_turret_model/traverse_model ==
  uh : Inport
  Th_x' : Inport  Port=2
  Integrator : Integrator
  Integrator1 : Integrator
  Sum : Sum  Inputs=|++
  calc_Mw_t : Subsystem
  calc_h'' : Subsystem
  calc_motor_torque : Subsystem
  h'' : Outport
  h' : Outport  Port=2
  h : Outport  Port=3
  h'_th_y : Outport  Port=4
  a_motor_torque : Outport  Port=5
  wires:
  Integrator/1 -> Sum/1, calc_Mw_t/1(h'), calc_motor_torque/1(h'), h'/1  "h'"
  uh/1 -> calc_motor_torque/2(uh)
  calc_motor_torque/1(motor_torque) -> a_motor_torque/1, calc_h''/2(motor_torque)
  calc_Mw_t/1(Mw_t) -> calc_h''/1(Mw_t)
  calc_h''/1(h'') -> h''/1, Integrator/1
  Integrator1/1 -> h/1  "h"
  Th_x'/1 -> Sum/2
  Sum/1 -> h'_th_y/1, Integrator1/1  "h'"

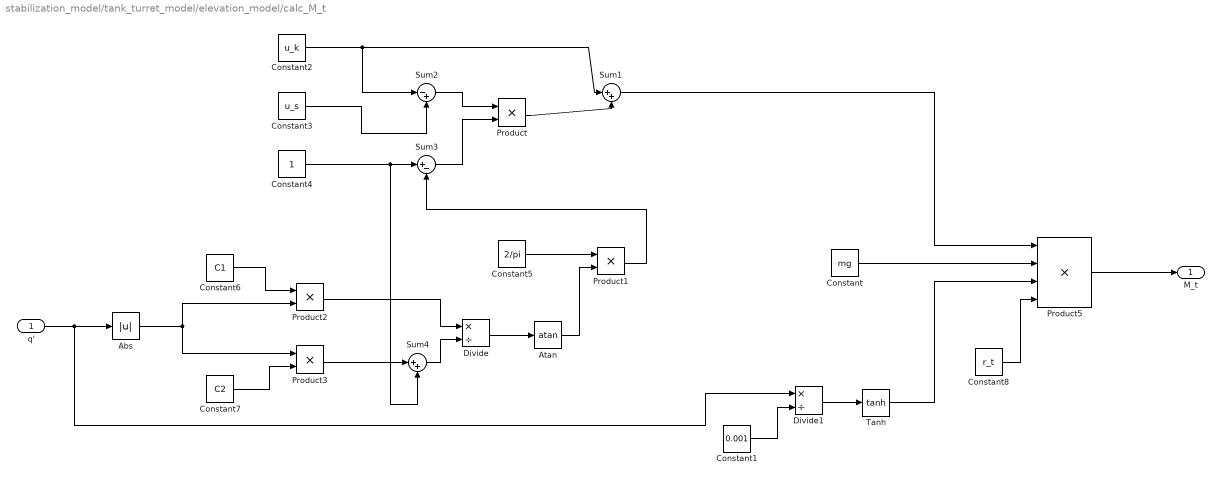
== system stabilization_model/tank_turret_model/elevation_model/calc_M_t ==
  q' : Inport
  Abs : Abs  SaturateOnIntegerOverflow=off
  Atan : Trigonometry  Operator=atan
  Constant : Constant  Value=mg
  Constant1 : Constant  Value=0.001
  Constant2 : Constant  Value=u_k
  Constant3 : Constant  Value=u_s
  Constant4 : Constant
  Constant5 : Constant  Value=2/pi
  Constant6 : Constant  Value=C1
  Constant7 : Constant  Value=C2
  Constant8 : Constant  Value=r_t
  Divide : Product  Inputs=*/
  Divide1 : Product  Inputs=*/
  Product{,1..3} (4 alike) : Product
  Product5 : Product  Inputs=4
  Sum1 : Sum  Inputs=|++
  Sum2 : Sum  Inputs=|-+
  Sum3 : Sum  Inputs=|+-
  Sum4 : Sum  Inputs=|++
  Tanh : Trigonometry  Operator=tanh
  M_t : Outport
  wires:
  Constant2/1 -> Sum1/1, Sum2/1
  Constant3/1 -> Sum2/2
  Sum2/1 -> Product/1
  Constant4/1 -> Sum4/2, Sum3/1
  Constant5/1 -> Product1/1
  Constant6/1 -> Product2/1
  q'/1 -> Divide1/1, Abs/1
  Abs/1 -> Product3/1, Product2/2
  Constant7/1 -> Product3/2
  Product3/1 -> Sum4/1
  Product2/1 -> Divide/1
  Sum4/1 -> Divide/2
  Divide/1 -> Atan/1
  Atan/1 -> Product1/2
  Product1/1 -> Sum3/2
  Sum3/1 -> Product/2
  Product/1 -> Sum1/2
  Sum1/1 -> Product5/1
  Constant/1 -> Product5/2
  Product5/1 -> M_t/1
  Tanh/1 -> Product5/3
  Constant1/1 -> Divide1/2
  Divide1/1 -> Tanh/1
  Constant8/1 -> Product5/4

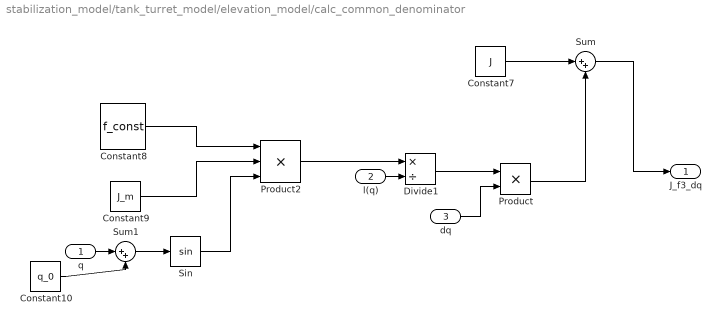
== system stabilization_model/tank_turret_model/elevation_model/calc_common_denominator ==
  q : Inport
  l(q) : Inport  Port=2
  dq : Inport  Port=3
  Constant10 : Constant  Value=q_0
  Constant7 : Constant  Value=J
  Constant8 : Constant  Value=f_const
  Constant9 : Constant  Value=J_m
  Divide1 : Product  Inputs=*/
  Product : Product
  Product2 : Product  Inputs=3
  Sin : Trigonometry
  Sum : Sum  Inputs=|++
  Sum1 : Sum  Inputs=|++
  J_f3_dq : Outport
  wires:
  Sum1/1 -> Sin/1
  Constant9/1 -> Product2/2
  Constant8/1 -> Product2/1
  Divide1/1 -> Product/1
  Constant10/1 -> Sum1/2
  Sin/1 -> Product2/3
  l(q)/1 -> Divide1/2
  Product2/1 -> Divide1/1
  q/1 -> Sum1/1
  Product/1 -> Sum/2
  dq/1 -> Product/2
  Constant7/1 -> Sum/1
  Sum/1 -> J_f3_dq/1

== system stabilization_model/tank_turret_model/elevation_model/calc_dq ==
  q : Inport
  l(q) : Inport  Port=2
  Constant : Constant  Value=l_1
  Constant1 : Constant  Value=l_2
  Constant2 : Constant  Value=q_0
  Divide : Product  Inputs=*/
  Product : Product
  Product1 : Product
  Sin : Trigonometry
  Sum : Sum  Inputs=|++
  dq : Outport
  wires:
  Sum/1 -> Sin/1
  Constant2/1 -> Sum/2
  Divide/1 -> dq/1
  Product/1 -> Product1/2
  Sin/1 -> Product1/1
  Constant1/1 -> Product/2
  Product1/1 -> Divide/1
  Constant/1 -> Product/1
  l(q)/1 -> Divide/2
  q/1 -> Sum/1

== system stabilization_model/tank_turret_model/elevation_model/calc_g1 ==
  J_f3_dq : Inport
  dq : Inport  Port=2
  Constant4 : Constant  Value=g1_const
  Divide : Product  Inputs=*/
  Product : Product
  g1 : Outport
  wires:
  Constant4/1 -> Product/1
  Product/1 -> Divide/1
  J_f3_dq/1 -> Divide/2
  Divide/1 -> g1/1
  dq/1 -> Product/2

== system stabilization_model/tank_turret_model/elevation_model/calc_g2 ==
  J_f3_dq : Inport
  Constant : Constant  Value=mgl
  Divide : Product  Inputs=*/
  g2 : Outport
  wires:
  J_f3_dq/1 -> Divide/2
  Constant/1 -> Divide/1
  Divide/1 -> g2/1

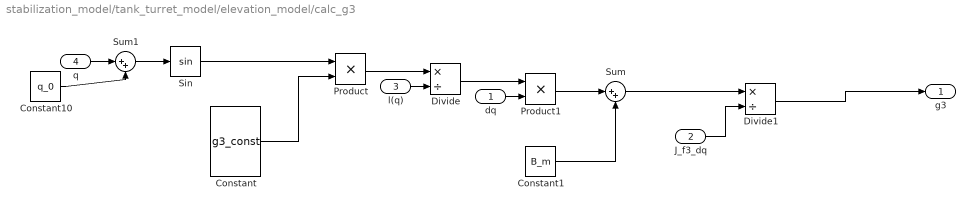
== system stabilization_model/tank_turret_model/elevation_model/calc_g3 ==
  dq : Inport
  J_f3_dq : Inport  Port=2
  l(q) : Inport  Port=3
  q : Inport  Port=4
  Constant : Constant  Value=g3_const
  Constant1 : Constant  Value=B_m
  Constant10 : Constant  Value=q_0
  Divide : Product  Inputs=*/
  Divide1 : Product  Inputs=*/
  Product : Product
  Product1 : Product
  Sin : Trigonometry
  Sum : Sum  Inputs=|++
  Sum1 : Sum  Inputs=|++
  g3 : Outport
  wires:
  Constant10/1 -> Sum1/2
  Sin/1 -> Product/1
  Product/1 -> Divide/1
  Sum1/1 -> Sin/1
  Product1/1 -> Sum/1
  Constant/1 -> Product/2
  Divide/1 -> Product1/1
  Constant1/1 -> Sum/2
  l(q)/1 -> Divide/2
  Sum/1 -> Divide1/1
  dq/1 -> Product1/2
  q/1 -> Sum1/1
  Divide1/1 -> g3/1
  J_f3_dq/1 -> Divide1/2

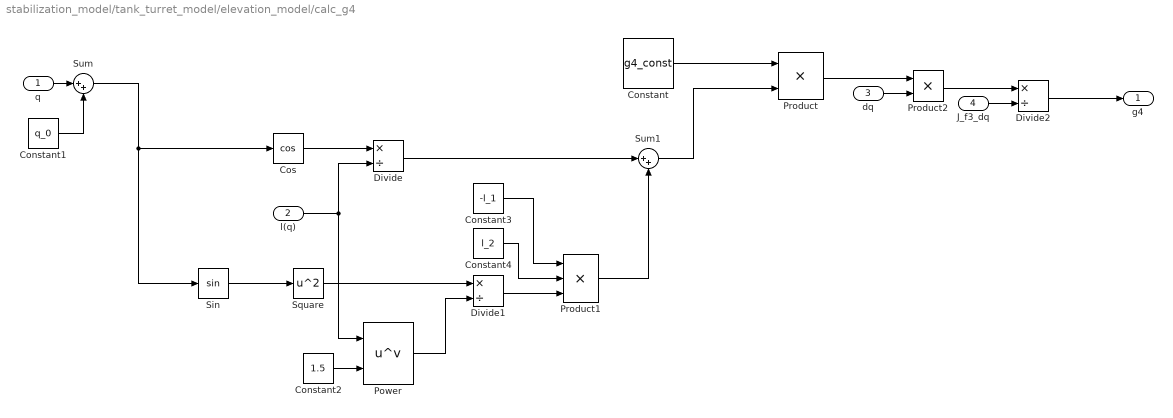
== system stabilization_model/tank_turret_model/elevation_model/calc_g4 ==
  q : Inport
  l(q) : Inport  Port=2
  dq : Inport  Port=3
  J_f3_dq : Inport  Port=4
  Constant : Constant  Value=g4_const
  Constant1 : Constant  Value=q_0
  Constant2 : Constant  Value=1.5
  Constant3 : Constant  Value=-l_1
  Constant4 : Constant  Value=l_2
  Cos : Trigonometry  Operator=cos
  Divide : Product  Inputs=*/
  Divide1 : Product  Inputs=*/
  Divide2 : Product  Inputs=*/
  Power : Math  Operator=pow
  Product : Product
  Product1 : Product  Inputs=3
  Product2 : Product
  Sin : Trigonometry
  Square : Math  Operator=square
  Sum : Sum  Inputs=|++
  Sum1 : Sum  Inputs=|++
  g4 : Outport
  wires:
  Sin/1 -> Square/1
  Constant/1 -> Product/1
  Power/1 -> Divide1/2
  Product1/1 -> Sum1/2
  Constant4/1 -> Product1/2
  Constant1/1 -> Sum/2
  Sum/1 -> Sin/1, Cos/1
  Constant3/1 -> Product1/1
  Cos/1 -> Divide/1
  Divide/1 -> Sum1/1
  Constant2/1 -> Power/2
  Divide1/1 -> Product1/3
  l(q)/1 -> Divide/2, Power/1
  Sum1/1 -> Product/2
  Square/1 -> Divide1/1
  q/1 -> Sum/1
  Product/1 -> Product2/1
  Divide2/1 -> g4/1
  Product2/1 -> Divide2/1
  dq/1 -> Product2/2
  J_f3_dq/1 -> Divide2/2

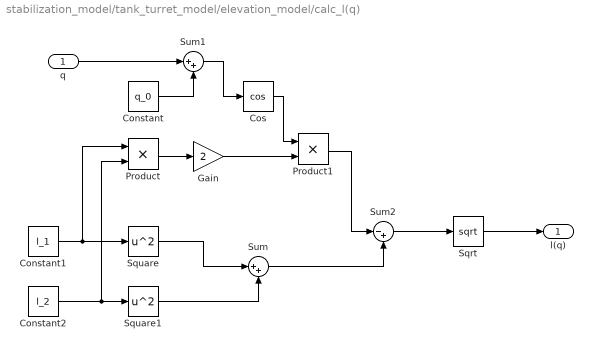
== system stabilization_model/tank_turret_model/elevation_model/calc_l(q) ==
  q : Inport
  Constant : Constant  Value=q_0
  Constant1 : Constant  Value=l_1
  Constant2 : Constant  Value=l_2
  Cos : Trigonometry  Operator=cos
  Gain : Gain  Gain=2
  Product : Product
  Product1 : Product
  Sqrt : Sqrt
  Square : Math  Operator=square
  Square1 : Math  Operator=square
  Sum : Sum  Inputs=|++
  Sum1 : Sum  Inputs=|++
  Sum2 : Sum  Inputs=|-+
  l(q) : Outport
  wires:
  Constant2/1 -> Product/2, Square1/1
  Sum/1 -> Sum2/2
  Product/1 -> Gain/1
  Square/1 -> Sum/1
  Constant1/1 -> Product/1, Square/1
  Product1/1 -> Sum2/1
  Constant/1 -> Sum1/2
  Square1/1 -> Sum/2
  Sum1/1 -> Cos/1
  Gain/1 -> Product1/2
  Cos/1 -> Product1/1
  q/1 -> Sum1/1
  Sum2/1 -> Sqrt/1
  Sqrt/1 -> l(q)/1

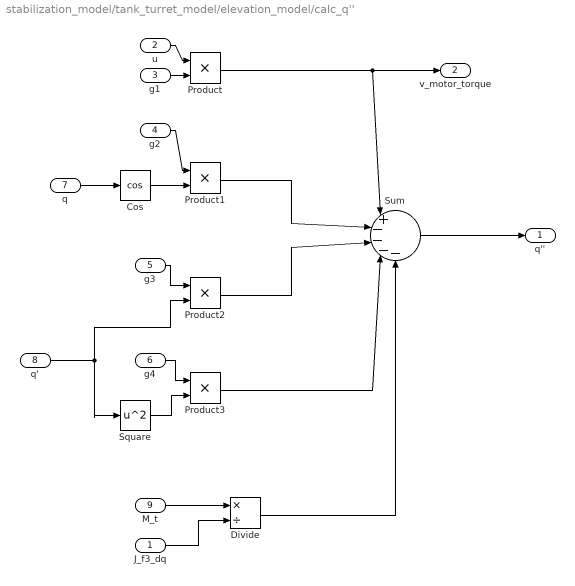
== system stabilization_model/tank_turret_model/elevation_model/calc_q'' ==
  J_f3_dq : Inport
  u : Inport  Port=2
  g1 : Inport  Port=3
  g2 : Inport  Port=4
  g3 : Inport  Port=5
  g4 : Inport  Port=6
  q : Inport  Port=7
  q' : Inport  Port=8
  M_t : Inport  Port=9
  Cos : Trigonometry  Operator=cos
  Divide : Product  Inputs=*/
  Product{,1..3} (4 alike) : Product
  Square : Math  Operator=square
  Sum : Sum  Inputs=|+----
  q'' : Outport
  v_motor_torque : Outport  Port=2
  wires:
  Product/1 -> Sum/1, v_motor_torque/1
  g1/1 -> Product/2
  Cos/1 -> Product1/2
  q/1 -> Cos/1
  g2/1 -> Product1/1
  g3/1 -> Product2/1
  g4/1 -> Product3/1
  u/1 -> Product/1
  q'/1 -> Product2/2, Square/1
  Product1/1 -> Sum/2
  Product2/1 -> Sum/3
  Product3/1 -> Sum/4
  Sum/1 -> q''/1
  Square/1 -> Product3/2
  M_t/1 -> Divide/1
  J_f3_dq/1 -> Divide/2
  Divide/1 -> Sum/5

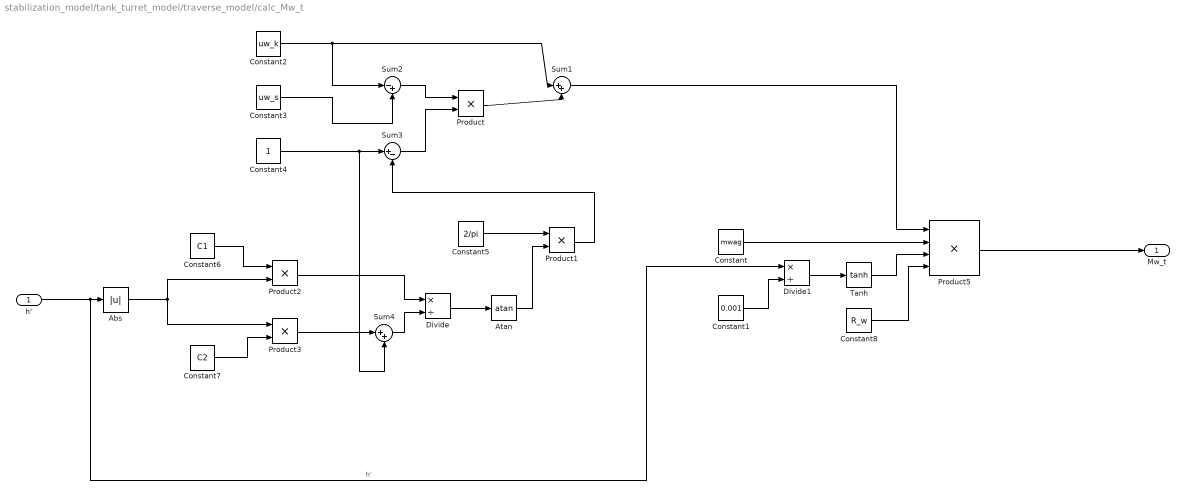
== system stabilization_model/tank_turret_model/traverse_model/calc_Mw_t ==
  h' : Inport
  Abs : Abs  SaturateOnIntegerOverflow=off
  Atan : Trigonometry  Operator=atan
  Constant : Constant  Value=mwag
  Constant1 : Constant  Value=0.001
  Constant2 : Constant  Value=uw_k
  Constant3 : Constant  Value=uw_s
  Constant4 : Constant
  Constant5 : Constant  Value=2/pi
  Constant6 : Constant  Value=C1
  Constant7 : Constant  Value=C2
  Constant8 : Constant  Value=R_w
  Divide : Product  Inputs=*/
  Divide1 : Product  Inputs=*/
  Product{,1..3} (4 alike) : Product
  Product5 : Product  Inputs=4
  Sum1 : Sum  Inputs=|++
  Sum2 : Sum  Inputs=|-+
  Sum3 : Sum  Inputs=|+-
  Sum4 : Sum  Inputs=|++
  Tanh : Trigonometry  Operator=tanh
  Mw_t : Outport
  wires:
  Constant2/1 -> Sum1/1, Sum2/1
  Constant3/1 -> Sum2/2
  Sum2/1 -> Product/1
  Constant4/1 -> Sum4/2, Sum3/1
  Constant5/1 -> Product1/1
  Constant6/1 -> Product2/1
  h'/1 -> Divide1/1, Abs/1  "h'"
  Abs/1 -> Product3/1, Product2/2
  Constant7/1 -> Product3/2
  Product3/1 -> Sum4/1
  Product2/1 -> Divide/1
  Sum4/1 -> Divide/2
  Divide/1 -> Atan/1
  Atan/1 -> Product1/2
  Product1/1 -> Sum3/2
  Sum3/1 -> Product/2
  Product/1 -> Sum1/2
  Sum1/1 -> Product5/1
  Constant/1 -> Product5/2
  Tanh/1 -> Product5/3
  Product5/1 -> Mw_t/1
  Divide1/1 -> Tanh/1
  Constant1/1 -> Divide1/2
  Constant8/1 -> Product5/4

== system stabilization_model/tank_turret_model/traverse_model/calc_h'' ==
  Mw_t : Inport
  motor_torque : Inport  Port=2
  Constant : Constant  Value=Jh
  Divide : Product  Inputs=*/
  Sum : Sum  Inputs=|+-
  h'' : Outport
  wires:
  Sum/1 -> Divide/1
  motor_torque/1 -> Sum/1
  Mw_t/1 -> Sum/2
  Constant/1 -> Divide/2
  Divide/1 -> h''/1

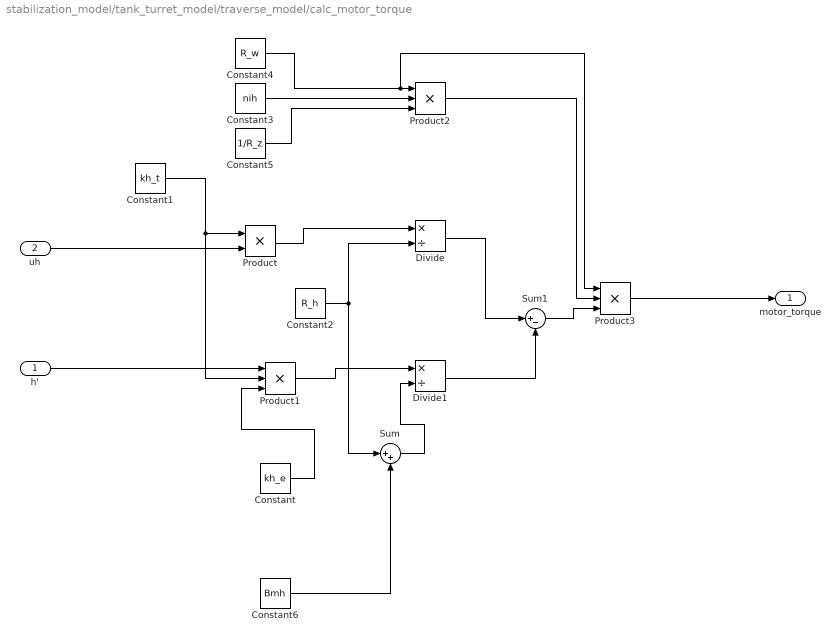
== system stabilization_model/tank_turret_model/traverse_model/calc_motor_torque ==
  h' : Inport
  uh : Inport  Port=2
  Constant : Constant  Value=kh_e
  Constant1 : Constant  Value=kh_t
  Constant2 : Constant  Value=R_h
  Constant3 : Constant  Value=nih
  Constant4 : Constant  Value=R_w
  Constant5 : Constant  Value=1/R_z
  Constant6 : Constant  Value=Bmh
  Divide : Product  Inputs=*/
  Divide1 : Product  Inputs=*/
  Product : Product
  Product1 : Product  Inputs=3
  Product2 : Product  Inputs=3
  Product3 : Product  Inputs=3
  Sum : Sum  Inputs=|++
  Sum1 : Sum  Inputs=|+-
  motor_torque : Outport
  wires:
  Constant2/1 -> Sum/1, Divide/2
  Constant1/1 -> Product1/2, Product/1
  Divide/1 -> Sum1/1
  Sum1/1 -> Product3/3
  Sum/1 -> Divide1/2
  Constant3/1 -> Product2/2
  Product/1 -> Divide/1
  Product1/1 -> Divide1/1
  Divide1/1 -> Sum1/2
  Product2/1 -> Product3/2
  Constant/1 -> Product1/3
  Constant4/1 -> Product3/1, Product2/1
  Constant5/1 -> Product2/3
  Constant6/1 -> Sum/2
  h'/1 -> Product1/1
  Product3/1 -> motor_torque/1
  uh/1 -> Product/2
